simulink model "single_FW_RL_high"  (R2022b)
settings: Solver=VariableStepAuto  StartTime=0.0  StopTime=00.04  RelTol=1e-3
libraries: spsDiodeLib x4, spsCurrentMeasurementLib x3, spsVoltageMeasurementLib x3, spsACVoltageSourceLib x1, spsSeriesRLCBranchLib x1, spspowerguiLib x1
settings Model: Creator=mroun  LastModifiedBy=mroun

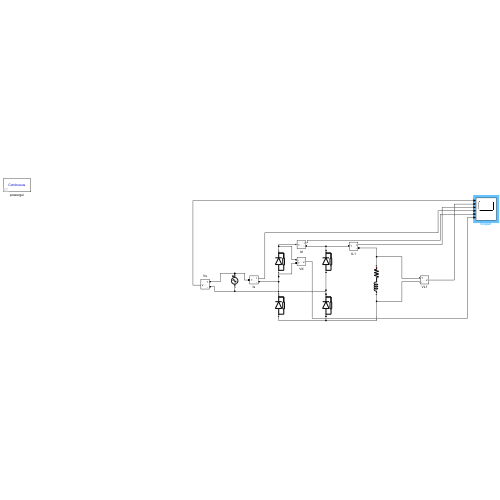
[thumbnail: Simulink's stored preview of the top-level diagram]
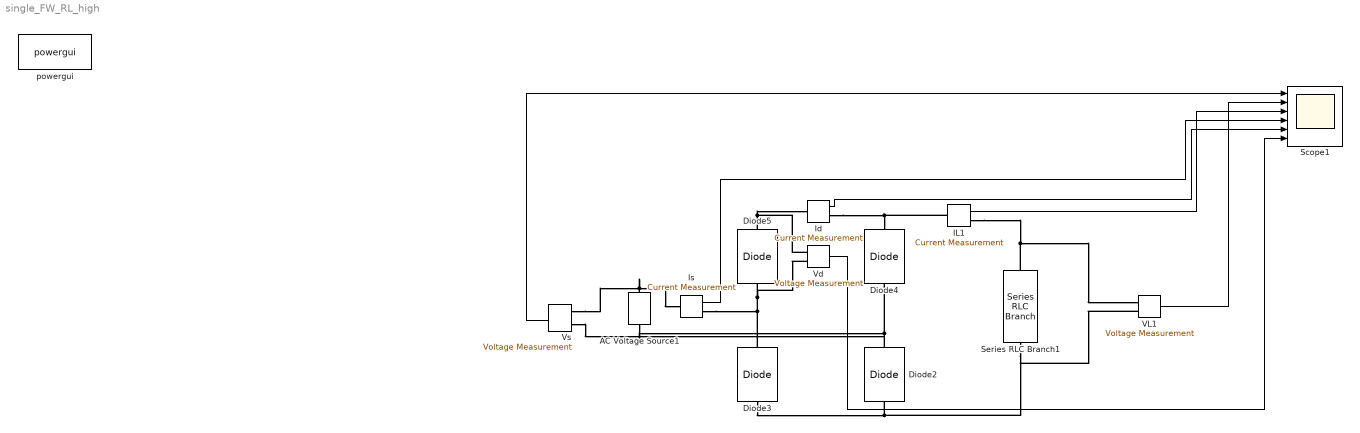
== system single_FW_RL_high ==
  AC Voltage Source1 : spsACVoltageSourceLib/AC Voltage Source  Amplitude=200  Phase=0  Frequency=50  SampleTime=0  Measurements=None  BusType=swing  Pref=10e3  Qref=0  Qmin=-inf  Qmax=+inf
  Diode{2..5} (4 alike) : spsDiodeLib/Diode  Ron=0.001  Lon=0  Vf=0.8  IC=0  UseSnubber=0  Rs=500  Cs=250e-9  Measurements=off
  IL1 : spsCurrentMeasurementLib/Current Measurement  PhasorSimulation=off  OutputType=Complex  PSBequivalent=0
  Id : spsCurrentMeasurementLib/Current Measurement  PhasorSimulation=off  OutputType=Complex  PSBequivalent=0
  Is : spsCurrentMeasurementLib/Current Measurement  PhasorSimulation=off  OutputType=Complex  PSBequivalent=0
  Scope1 : Scope  NumInputPorts=6
  Series RLC Branch1 : spsSeriesRLCBranchLib/Series RLC Branch  LConnTagsString=__new0  RConnTagsString=__new0  BranchType=RL  Resistance=10  Inductance=.2  SetiL0=off  InitialCurrent=2  Capacitance=1e-6  Setx0=off  InitialVoltage=0  Measurements=None
  VL1 : spsVoltageMeasurementLib/Voltage Measurement  PhasorSimulation=off  OutputType=Complex  PSBequivalent=0
  Vd : spsVoltageMeasurementLib/Voltage Measurement  PhasorSimulation=off  OutputType=Complex  PSBequivalent=0
  Vs : spsVoltageMeasurementLib/Voltage Measurement  PhasorSimulation=off  OutputType=Complex  PSBequivalent=0
  powergui : spspowerguiLib/powergui  Priority=1  SimulationMode=Continuous  SampleTime=50e-6  frequency=60  Iterations=50  frequencyindice=50  Pbase=100e6  ErrMax=1e-4  UnitsV=kV  UnitsW=MW  buscounter=0  FunctionMessages=off  echomessages=off  EnableUseOfTLC=off  CurrentSourceSwitches=off  DisableSnubberDevices=off  DisableRonSwitches=off  DisableVfSwitches=off  DisplayEquations=off  AutomaticDiscreteSolvers=off  SolverType=Tustin/Backward Euler (TBE)  Interpol=off  ExternalGateDelay=off  methode=off  Ts=100  x0status=blocks  SPID=on  SwTol=0  HookPort=off  NonlinearTolerance=1e-4  nMaxIteration=100  ContinueOnMaxIteration=off  RestoreLinks=warning  ResistiveCurrentMeasurement=off  Frange=[0:2:500]  Ylog=off  Xlog=on  ShowGrid=off  save=off  variable=ZData  structure=0  ZoomFFT=off  StartTime=0.0  cycles=1  DisplayStyle=1  fundamental=60  FreqAxis=off  MaxFrequency=1000  frequencyindicesteady=1  RmsSteady=1  display=off
  wires:
  VL1/1 -> Scope1/2
  IL1/1 -> Scope1/3
  Vs/1 -> Scope1/1
  Is/1 -> Scope1/4
  Id/1 -> Scope1/5
  Vd/1 -> Scope1/6
  connections:
  Diode3/RConn1 -- Vd/LConn1 -- Diode5/LConn1 -- Is/RConn1
  Diode2/RConn1 -- AC Voltage Source1/LConn1 -- Vs/LConn2 -- Diode4/LConn1
  IL1/LConn1 -- Id/RConn1 -- Diode4/RConn1
  Diode3/LConn1 -- VL1/LConn2 -- Series RLC Branch1/RConn1 -- Diode2/LConn1
  Series RLC Branch1/LConn1 -- IL1/RConn1 -- VL1/LConn1
  AC Voltage Source1/RConn1 -- Is/LConn1 -- Vs/LConn1
  Diode5/RConn1 -- Vd/LConn2 -- Id/LConn1
